simulink model "base"  (Simulink 8.7)
settings: Solver=ode1  StartTime=0.0  StopTime=inf  FixedStep=0.001  RelTol=1e-3
PostLoadFcn:
  | , if any(exist('dsrtsu_mdlpostloadfcn', 'file') == [2, 3, 6]), try dsrtsu_mdlpostloadfcn('Execute', bdroot); catch fprintf('Error in PostLoadFcn (dsrtsu_mdlpostloadfcn) for model "%s":\n %s\n', bdroot, lasterr); end, end,
libraries: rtiethernetlib x4, dsextras x1
settings Model: DSRTSU_INTERNAL_RTI_VER=480  DSRTSU_INTERNAL_RTI_TYPE=rti1007  DSRTSU_INTERNAL_RTIFPGA=70  Creator=murakami  LastModifiedBy=higo
settings DataIOCC: SignalLoggingSaveFormat=ModelDataLogs
settings OptimizationCC: BlockReduction=off  ExpressionDepthLimit=2147483647  InitFltsAndDblsToZero=on
settings DebuggingCC: AlgebraicLoopMsg=none  SaveWithParameterizedLinksMsg=none  SignalResolutionControl=TryResolveAllWithWarning  SolverPrmCheckMsg=warning  InheritedTsInSrcMsg=none  MultiTaskDSMMsg=warning  MultiTaskCondExecSysMsg=none  FcnCallInpInsideContextMsg=UseLocalSettings  UnconnectedInputMsg=none  UnconnectedOutputMsg=none  UnconnectedLineMsg=none  StateNameClashWarn=warning
settings HardwareCC: ProdLargestAtomicInteger=Integer  ProdLargestAtomicFloat=Float  ProdIntDivRoundTo=Zero  ProdEndianess=BigEndian  ProdHWDeviceType=Custom Processor->Custom  TargetIntDivRoundTo=Zero  TargetEndianess=BigEndian  TargetHWDeviceType=Custom Processor->Custom
settings RTWCC: SystemTargetFile=rti1007.tlc  MakeCommand=make_rti  TemplateMakefile=rti1007.tmf  Description=dSPACE DS1007 Hardware Platform
settings STFCustomTargetCC: ParMdlRefBuildCompliant=on  SystemTargetFile=rti1007.tlc
settings GRTTargetCC: CompOptLevelCompliant=off  ConcurrentExecutionCompliant=off  GeneratePreprocessorConditionals=Use local settings  CombineOutputUpdateFcns=off  MatFileLogging=off  CPPClassGenCompliant=off  GRTInterface=on  UseToolchainInfoCompliant=off  ExtModeMexFile=noextcomm
settings CustomProperty: DataType=RTWOptions_EnumType_C__Program Files_dSPACE RCPHIL 2016-A_MATLAB_RTI_RTI1007_TLC_rti1007_1InitialSimState  Value=RUN
settings EnumStrPairs: String=RUN

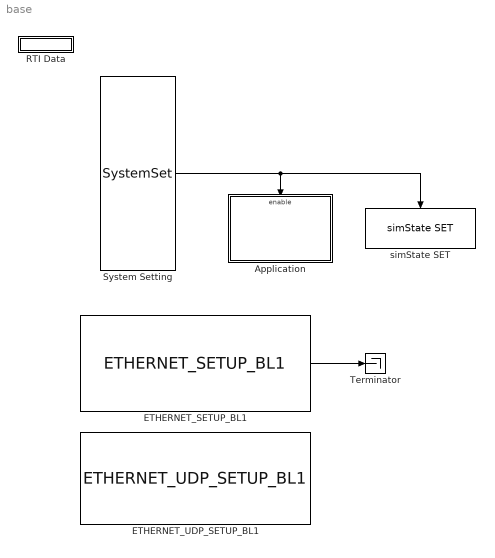
== system base ==
  Application : Subsystem  TreatAsAtomicUnit=on
  ETHERNET_SETUP_BL1 : rtiethernetlib/ETHERNET_SETUP_BL1  DSProperties=struct('RTI',struct('Version',uint32(2),'BlockType',struct('isSLSource',uint8(0),'isSLSink',uint8(0),'isHWSource',uint8(0),'isHWSink',uint8(0),'isSetup',uint8(1),'isInline',uint8(1),'isNonInline',uint8(0),'isInterrupt',uint8(0),'isChannelwise',uint8(0)),'IOBoardType','DSETHERNET','UnitType','ETHERNET','Identifier','SETUP','DialogType','ML','BlockSet','RTIETHERNET','SlaveProcessor','NONE'))  RTIBlockInterface=struct('OutputPortsWidth',int32([2 1 1 4]),'OutputPortsActive',[1 0 0 0],'OutputPortsName',{{['Link Status'],['Watchdog Status'],['DHCP Status'],['Local IP']}},'OutputPortsDataType',{{'SS_UINT32','SS_UINT32','SS_UINT32','SS_UINT8'}},'InitLevel',3,'IconTransparency','on','BlockDisplay',{{['Ethernet Setup\n\nLocal IP: 10.1.196.179'],'left'}},'DialogFcn','rtiethernetsetupgui','BlockName',struct('Token',{{'ETHERNET_SETUP_BL1'}}))  RTIBlockParameters=struct('DHCPserverMode',{{0,'OFF',[0 1]}},'LocalIpNum1',{{'10','OFF',[0 255]}},'LocalIpNum2',{{'1','OFF',[0 255]}},'LocalIpNum3',{{'196','OFF',[0 255]}},'LocalIpNum4',{{'179','OFF',[0 255]}},'SubnetMaskNum1',{{'255','OFF',[0 255]}},'SubnetMaskNum2',{{'255','OFF',[0 255]}},'SubnetMaskNum3',{{'255','OFF',[0 255]}},'SubnetMaskNum4',{{'0','OFF',[0 255]}},'GatewayNum1',{{'0','OFF',[0 255]}},'GatewayNum2',{{'0','OFF',[0 255]}},'GatewayNum3',{{'0','OFF',[0 255]}},'GatewayNum4',{{'0','OFF',[0 255]}},'LinkStatusOutPortMode',{{1,'OFF',[0 1]}},'NumOfEthConnectors',{{2,'ON',[1 16]}},'WatchdogStatusOutPortMode',{{0,'OFF',[0 1]}},'LocalIpOutPortMode',{{0,'OFF',[0 1]}},'IpAndSubmaskCheck',{{int32(1),'OFF',[0 1]}},'TLCFileName',{{'rtiethernetsetup','OFF',[]}})  RTISFcnParameters=struct('DHCPserverMode','int32','LocalIpNum1','uint8','LocalIpNum2','uint8','LocalIpNum3','uint8','LocalIpNum4','uint8','SubnetMaskNum1','uint8','SubnetMaskNum2','uint8','SubnetMaskNum3','uint8','SubnetMaskNum4','uint8','GatewayNum1','uint8','GatewayNum2','uint8','GatewayNum3','uint8','GatewayNum4','uint8','LinkStatusOutPortMode','int32','NumOfEthConnectors','int32','WatchdogStatusOutPortMode','int32','LocalIpOutPortMode','int32','TLCFileName','char')  RTIBlockParaDefault=struct('DHCPserverMode',0,'LocalIpNum1',192,'LocalIpNum2',168,'LocalIpNum3',140,'LocalIpNum4',6,'SubnetMaskNum1',255,'SubnetMaskNum2',255,'SubnetMaskNum3',255,'SubnetMaskNum4',0,'GatewayNum1',0,'GatewayNum2',0,'GatewayNum3',0,'GatewayNum4',0,'LinkStatusOutPortMode',1,'NumOfEthConnectors',3,'WatchdogStatusOutPortMode',0,'LocalIpOutPortMode',0,'IpAndSubmaskCheck',1,'TLCFileName','rtiethernetsetup')
  ETHERNET_UDP_SETUP_BL1 : rtiethernetlib/ETHERNET_UDP_SETUP_BL1  DSProperties=struct('RTI',struct('Version',uint32(2),'BlockType',struct('isSLSource',uint8(1),'isSLSink',uint8(1),'isHWSource',uint8(0),'isHWSink',uint8(0),'isSetup',uint8(0),'isInline',uint8(1),'isNonInline',uint8(0),'isInterrupt',uint8(0),'isChannelwise',uint8(0)),'IOBoardType','DSETHERNET','UnitType','UDP','Identifier','SETUPUDP','DialogType','ML','BlockSet','RTIETHERNET','SlaveProcessor','NONE'))  RTIBlockInterface=struct('OutputPortsWidth',int32(2),'OutputPortsActive',0,'OutputPortsName',{{['RX Dropped Frames']}},'OutputPortsDataType',{{'SS_DOUBLE'}},'InputPortsWidth',int32([4 1]),'InputPortsActive',int32([0 0]),'InputPortsName',{{['RX Remote IP Filter'],['RX Remote Port Filter']}},'InputPortsDataType',{{'SS_UINT8','SS_UINT16'}},'RWork',{{{'RX_DROPPED_FRAMES',uint32(2)}}},'InitLevel',3,'IconTransparency','on','BlockDisplay',{{['Ethernet UDP/IP\nSetup\n\nSocket ID: 0'],'center'}},'DialogFcn','rtiethernetsetupudpgui','BlockName',struct('Token',{{'ETHERNET_UDP_SETUP_BL1'}}))  RTIBlockParameters=struct('SocketId',{{0,'OFF',[]}},'EnableSocketBind',{{1,'OFF',[0 1]}},'AcceptAnyRxRemoteIp',{{1,'OFF',[0 1]}},'RxRemoteIpNum1',{{'10','OFF',[0 255]}},'RxRemoteIpNum2',{{'1','OFF',[0 255]}},'RxRemoteIpNum3',{{'196','OFF',[0 255]}},'RxRemoteIpNum4',{{'18','OFF',[0 255]}},'EnableDynamicRxRemoteIpFilter',{{0,'OFF',[0 1]}},'AcceptAnyRxRemotePort',{{1,'OFF',[0 1]}},'RxRemotePort',{{'49002','OFF',[1 65535]}},'EnableDynamicRxRemotePortFilter',{{0,'OFF',[0 1]}},'TxRemoteIpNum1',{{'10','OFF',[0 255]}},'TxRemoteIpNum2',{{'1','OFF',[0 255]}},'TxRemoteIpNum3',{{'196','OFF',[0 255]}},'TxRemoteIpNum4',{{'178','OFF',[0 255]}},'TxRemotePort',{{'52001','OFF',[1 65535]}},'SpecifyLocalPort',{{1,'OFF',[0 1]}},'LocalPort',{{'50006','OFF',[1 65535]}},'InterruptMode',{{0,'OFF',[0 1]}},'RxDroppedFramesOutPortMode',{{0,'OFF',[0 1]}},'RemoteIpNumCheck',{{0,'OFF',[0 1]}},'RemotePortCheck',{{0,'OFF',[0 1]}},'LocalPortCheck',{{1,'OFF',[0 1]}},'DHCPserverModeEnabled',{{0,'OFF',[0 1]}},'TLCFileName',{{'rtiethernetsetupudp','OFF',[]}})  RTISFcnParameters=struct('SocketId','double','EnableSocketBind','int32','AcceptAnyRxRemoteIp','int32','RxRemoteIpNum1','uint8','RxRemoteIpNum2','uint8','RxRemoteIpNum3','uint8','RxRemoteIpNum4','uint8','EnableDynamicRxRemoteIpFilter','int32','AcceptAnyRxRemotePort','int32','RxRemotePort','uint16','EnableDynamicRxRemotePortFilter','int32','TxRemoteIpNum1','uint8','TxRemoteIpNum2','uint8','TxRemoteIpNum3','uint8','TxRemoteIpNum4','uint8','TxRemotePort','uint16','SpecifyLocalPort','int32','LocalPort','uint16','InterruptMode','int32','RxDroppedFramesOutPortMode','int32','DHCPserverModeEnabled','int32','TLCFileName','char')  RTIBlockParaDefault=struct('SocketId',-1,'EnableSocketBind',1,'AcceptAnyRxRemoteIp',1,'RxRemoteIpNum1',0,'RxRemoteIpNum2',0,'RxRemoteIpNum3',0,'RxRemoteIpNum4',0,'EnableDynamicRxRemoteIpFilter',0,'AcceptAnyRxRemotePort',1,'RxRemotePort',49002,'EnableDynamicRxRemotePortFilter',0,'TxRemoteIpNum1',0,'TxRemoteIpNum2',0,'TxRemoteIpNum3',0,'TxRemoteIpNum4',0,'TxRemotePort',49002,'SpecifyLocalPort',0,'LocalPort',49001,'InterruptMode',0,'RxDroppedFramesOutPortMode',0,'RemoteIpNumCheck',0,'RemotePortCheck',0,'LocalPortCheck',0,'DHCPserverModeEnabled',0,'TLCFileName','rtiethernetsetupudp')
  RTI Data : Subsystem  Tag=struct('RTIDataServer',struct('RTIDataServerVs','2','RTIModelDescription','struct(''main'',''base'',''sub'','''',''isMp'',0)'))  LoadFcn="if exist('rtidc'), try,  rtidc('DataHostBlockClbLoad', gcbh); catch, disp(['Warning: ''LoadFcn'' for RTI Data block failed: ' lasterr]); end, end,"  mask(RTI_DATA_HOST){}
      mask help:
      | RTI Data Block.
      | This block is used by RTI to store internal model-dependent data.
      | Please keep this block on the root level of the model. Deleting this block will result in data loss.
      |
      | NEVER DELETE OR COPY THIS BLOCK!
      settings: CopyFcn="if exist('rtidc'), try,  rtidc('DataHostBlockClbCopy', gcbh); catch, disp(['Warning: ''CopyFcn'' for RTI Data block failed: ' lasterr]); end, end,"  DeleteFcn="if exist('rtidc'), try,  rtidc('DataHostBlockClbDelete', gcbh); catch, disp(['Warning: ''DeleteFcn'' for RTI Data block failed: ' lasterr]); end, end,"  ModelCloseFcn="if exist('rtidc'), try,  rtidc('DataHostBlockClbModelClose', gcbh); catch, disp(['Warning: ''ModelCloseFcn'' for RTI Data block failed: ' lasterr]); end, end,"  PreSaveFcn="if exist('rtidc'), try,  rtidc('DataHostBlockClbPreSave', gcbh); catch, disp(['Warning: ''PreSaveFcn'' for RTI Data block failed: ' lasterr]); end, end,"  PostSaveFcn="if exist('rtidc'), try,  rtidc('DataHostBlockClbPostSave', gcbh); catch, disp(['Warning: ''PostSaveFcn'' for RTI Data block failed: ' lasterr]); end, end,"  NameChangeFcn="if exist('rtidc'), try,  rtidc('DataHostBlockClbNameChange', gcbh); catch, disp(['Warning: ''NameChangeFcn'' for RTI Data block failed: ' lasterr]); end, end,"
      mask Help:
      | RTI Data Block.
      | This block is used by RTI to store internal model-dependent data.
      | Please keep this block on the root level of the model. Deleting this block will result in data loss.
      | 
      | NEVER DELETE OR COPY THIS BLOCK!
      mask Display:
      | text(0.5, 0.5, 'RTI Data', 'HorizontalAlignment', 'center');
      | plot([1 0]);
  System Setting : S-Function  FunctionName=SystemSet  SFunctionDeploymentMode=off  EnableBusSupport=off
  Terminator : Terminator
  simState SET : dsextras/simState SET  TriggerPort=falling  EnablePort=none  SimStateMode=STOP  TLCFileName=rti_simstate_set  Reserved1=[]  Reserved2=[]  Reserved3=[]  Reserved4=[]  DSProperties=struct('RTI',struct('Version',uint32(1),'BlockType',struct('isSLSource',uint8(1),'isSLSink',uint8(0),'isHWSource',uint8(0),'isHWSink',uint8(0),'isSetup',uint8(0),'isInline',uint8(1),'isNonInline',uint8(0),'isInterrupt',uint8(0),'isChannelwise',uint8(0)),'IOBoardType','EXTRAS','UnitType','SIMSTATESET','Identifier','SIMSTATESET','DialogType','SL','BlockSet','NONE','SlaveProcessor','NONE'))  RTIBlockInterface=struct('OutputPortsWidth',int32(0),'BlockDisplay',{{['simState STOP'],'center'}},'IconTransparency','on','InitLevel',2,'BlockName',struct('Token',{{['simState SET']}}),'TriggerPort',{{'falling'}},'EnablePort',{{'none'}},'MaskDescription',['Set simState to the specified value when the block is executed.'])  RTIBlockParameters=struct('TriggerPort',{{3,'OFF',[]}},'EnablePort',{{1,'OFF',[]}},'SimStateMode',{{3,'OFF',[]}},'TLCFileName',{{'rti_simstate_set','OFF',[]}})  RTISFcnParameters=struct('TriggerPort','double','EnablePort','double','SimStateMode','char','TLCFileName','char')  RTIBlockParaDefault=struct('TriggerPort',2,'EnablePort',1,'SimStateMode',1,'TLCFileName','rti_simstate_set')
  wires:
  ETHERNET_SETUP_BL1/1 -> Terminator/1
  System Setting/1 -> Application/Enable, simState SET/Trigger

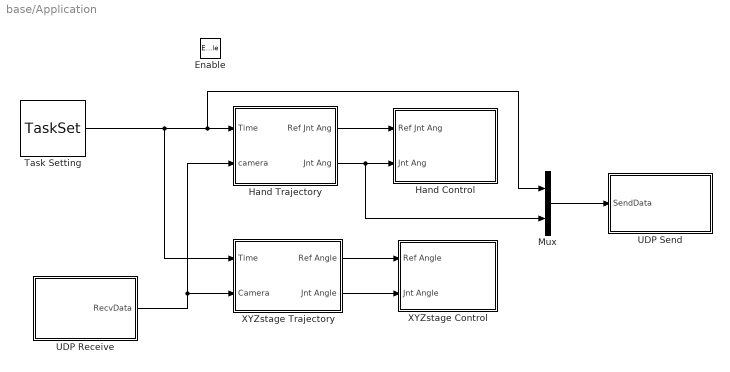
== system base/Application ==
  Enable : EnablePort  StatesWhenEnabling=reset
  Hand Control : Subsystem
  Hand Trajectory : Subsystem
  Mux : Mux  Inputs=2
  Task Setting : S-Function  FunctionName=TaskSet  SFunctionDeploymentMode=off  EnableBusSupport=off
  UDP Receive : Subsystem
  UDP Send : Subsystem
  XYZstage Control : Subsystem
  XYZstage Trajectory : Subsystem
  wires:
  Hand Trajectory/1(Ref Jnt Ang) -> Hand Control/1(Ref Jnt Ang)
  Hand Trajectory/2(Jnt Ang) -> Mux/2, Hand Control/2(Jnt Ang)
  Task Setting/1 -> XYZstage Trajectory/1(Time), Mux/1, Hand Trajectory/1(Time)
  UDP Receive/1(RecvData) -> XYZstage Trajectory/2(Camera), Hand Trajectory/2(camera)
  XYZstage Trajectory/1(Ref Angle) -> XYZstage Control/1(Ref Angle)
  XYZstage Trajectory/2(Jnt Angle) -> XYZstage Control/2(Jnt Angle)
  Mux/1 -> UDP Send/1(SendData)

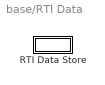
== system base/RTI Data ==
  RTI Data Store : Subsystem  Tag="struct('private',struct('version',struct('dsVer',uint32(2)),'access',struct('modified',['23-Jul-2018 20:42:30'],'type','Model','isPerm',1)),'public',struct('main',struct('data',[]),'sub',struct('name',{{'base'}},'data',{{struct('TH',struct('thTaskInfo',struct('taskType',{'TIMER','HWINT','TMRINT','SWINT','GLINT'},'tasksNumOf',{1,0,0,0,0},'srcIds',{{'TIMERA'},{},{},{},{}},'taskNames',{{['Timer Task 1']},{},{},{},{}})),'th_tc',struct('dataType','TASK','taskGroupId','','taskGroupList',{{}},'taskSchedulingPolicy','FCFS','taskType','TIMER','blkh',-1,'srcId','TIMERA','srcSgnName',['Timer A interrupt'],'srcCpuName','','taskName',['Timer Task 1  [0.001] s'],'taskNameDisplayExt','','smplTime',0.001,'smplTimeOffs',0,'hasFixedPriority',0,'priority',1,'hasFixedOvc',0,'ovcType',1,'ovcMax',1),'tc_th',struct('dataType','TASK','taskGroupId','','taskGroupList',{{}},'taskSchedulingPolicy','FCFS','taskType','TIMER','blkh',-1,'srcId','TIMERA','srcSgnName',['Timer A interrupt'],'srcCpuName','','taskName',['Timer Task 1  [0.001] s'],'taskNameDisplayExt','','smplTime',0.001,'smplTimeOffs',0,'hasFixedPriority',0,'priority',1,'hasFixedOvc',0,'ovcType',1,'ovcMax',1))}})))"  mask(RTI_DATA_STORE){}
      mask help:
      | RTI Data Store Block. This block is used by RTI to store internal model dependent data. Deleting this block will result in data loss.
      |
      | NEVER DELETE, COPY, OR MODIFY THIS BLOCK!
      mask Help:
      | RTI Data Store Block. This block is used by RTI to store internal model dependent data. Deleting this block will result in data loss.
      | 
      | NEVER DELETE, COPY, OR MODIFY THIS BLOCK!
      mask Display: text(0.5, 0.5, ' ', 'HorizontalAlignment', 'center');

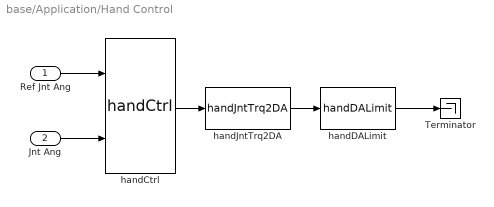
== system base/Application/Hand Control ==
  Ref Jnt Ang : Inport
  Jnt Ang : Inport  Port=2
  Terminator : Terminator
  handCtrl : S-Function  FunctionName=handCtrl  SFunctionDeploymentMode=off  EnableBusSupport=off
  handDALimit : S-Function  FunctionName=handDALimit  SFunctionDeploymentMode=off  EnableBusSupport=off
  handJntTrq2DA : S-Function  FunctionName=handJntTrq2DA  SFunctionDeploymentMode=off  EnableBusSupport=off
  wires:
  Jnt Ang/1 -> handCtrl/2
  Ref Jnt Ang/1 -> handCtrl/1
  handCtrl/1 -> handJntTrq2DA/1
  handJntTrq2DA/1 -> handDALimit/1
  handDALimit/1 -> Terminator/1

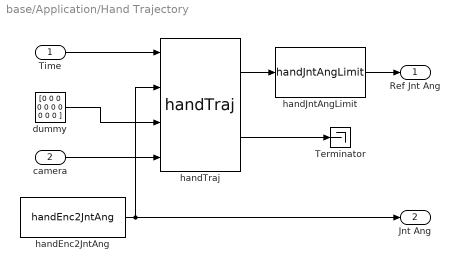
== system base/Application/Hand Trajectory ==
  Time : Inport
  camera : Inport  Port=2
  Terminator : Terminator
  dummy : Constant  Value=[0 0 0 0 0 0 0 0 0 0 ]
  handEnc2JntAng : S-Function  FunctionName=handEnc2JntAng  SFunctionDeploymentMode=off  EnableBusSupport=off
  handJntAngLimit : S-Function  FunctionName=handJntAngLimit  SFunctionDeploymentMode=off  EnableBusSupport=off
  handTraj : S-Function  FunctionName=handTraj  SFunctionDeploymentMode=off  EnableBusSupport=off
  Ref Jnt Ang : Outport
  Jnt Ang : Outport  Port=2
  wires:
  Time/1 -> handTraj/1
  handEnc2JntAng/1 -> handTraj/2, Jnt Ang/1
  handTraj/1 -> handJntAngLimit/1
  handJntAngLimit/1 -> Ref Jnt Ang/1
  handTraj/2 -> Terminator/1
  dummy/1 -> handTraj/3
  camera/1 -> handTraj/4

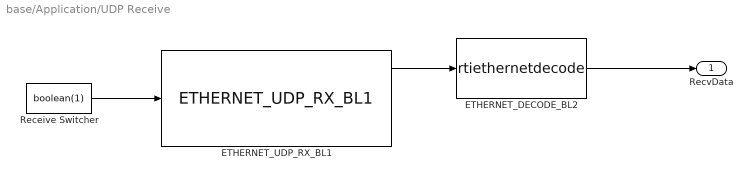
== system base/Application/UDP Receive ==
  ETHERNET_DECODE_BL2 : S-Function  FunctionName=rtiethernetdecode  Parameters=byteordering,offset,auto_offset,datatype,one_datatype,sampletime  SFunctionDeploymentMode=off  EnableBusSupport=off  mask(Ethernet Decode){byteordering=Little endian (Intel), offset=[0], auto_offset=on, datatype=9, one_datatype=on, sampletime=-1}
      mask prompts: byteordering "Byte ordering:"; offset "Offset (bytes):"; auto_offset "Auto offset"; one_datatype "One datatype only"
      mask help:
      | Converts a byte input data stream into the specified datatypes on the output port.
      |
      | Datatype codes:
      | BOOLEAN:  1   //   INT8:      2   //   UINT8:    3
      | INT16  :     4   //   UINT16:  5   //   INT32:     6
      | UINT32 :    7   //   FLOAT:    8   //   DOUBLE:  9
      mask Help: To get further information on this block, refer to the RTI Ethernet blockset documentation.
      mask TypeOptions byteordering: Big endian (Motorola) | Little endian (Intel)
      mask Callback auto_offset: rtiethernetfcnlib('EnableEnDecodeGuiControl', gcbh, 'auto_offset', 2)
      mask Display: text(0.5,0.5, 'Ethernet\nDecode', 'HorizontalAlignment', 'center')
  ETHERNET_UDP_RX_BL1 : rtiethernetlib/ETHERNET_UDP_RX_BL1  DSProperties=struct('RTI',struct('Version',uint32(1),'BlockType',struct('isSLSource',uint8(1),'isSLSink',uint8(1),'isHWSource',uint8(0),'isHWSink',uint8(1),'isSetup',uint8(0),'isInline',uint8(1),'isNonInline',uint8(0),'isInterrupt',uint8(0),'isChannelwise',uint8(0)),'IOBoardType','DSETHERNET','UnitType','UDP','Identifier','RXUDP','DialogType','ML','BlockSet','RTIETHERNET','SlaveProcessor','NONE'))  RTIBlockInterface=struct('OutputPortsWidth',int32([112 1 1 1 4 1]),'OutputPortsActive',[1 1 1 0 0 0],'OutputPortsName',{{'Data','Status',['Received Frames'],['Received Bytes'],['Remote IP'],['Remote Port']}},'OutputPortsDataType',{{'SS_UINT8','SS_UINT32','SS_DOUBLE','SS_UINT32','SS_UINT8','SS_UINT16'}},'InputPortsWidth',int32(1),'InputPortsActive',1,'InputPortsName',{{'Enable'}},'InputPortsDataType',{{'SS_BOOLEAN'}},'RWork',{{{'RECEIVED_FRAMES',uint32(1)}}},'InitLevel',3,'IconTransparency','on','BlockDisplay',{{['Ethernet UDP/IP\nRX\n\nSocket ID: 0'],'center'}},'DialogFcn','rtiethernetrxudpgui','BlockName',struct('Token',{{'ETHERNET_UDP_RX_BL1'}}))  RTIBlockParameters=struct('SocketIdIndex',{{2,'OFF',[1 2]}},'SocketId',{{0,'OFF',[-1 inf]}},'RemoteIp',{{['<NOT AVAILABLE>'],'OFF',[]}},'RemotePort',{{['<NOT AVAILABLE>'],'OFF',[]}},'LocalPort',{{50006,'OFF',[]}},'FrameSize',{{'112','OFF',[1 65507]}},'EnableVariableFrameSize',{{0,'OFF',[0 1]}},'VariableFrameSizeMode',{{1,'OFF',[1 2]}},'InterruptMode',{{0,'OFF',[0 1]}},'RemoteIpOutPortMode',{{0,'OFF',[0 1]}},'RemotePortOutPortMode',{{0,'OFF',[0 1]}},'TLCFileName',{{'rtiethernetrxudp','OFF',[]}})  RTISFcnParameters=struct('SocketIdIndex','int32','SocketId','double','FrameSize','uint16','EnableVariableFrameSize','int32','VariableFrameSizeMode','int32','InterruptMode','int32','RemoteIpOutPortMode','int32','RemotePortOutPortMode','int32','TLCFileName','char')  RTIBlockParaDefault=struct('SocketIdIndex',1,'SocketId',-1,'RemoteIp',['<NOT AVAILABLE>'],'RemotePort',['<NOT AVAILABLE>'],'LocalPort',['<NOT AVAILABLE>'],'FrameSize',1024,'EnableVariableFrameSize',0,'VariableFrameSizeMode',1,'InterruptMode',0,'RemoteIpOutPortMode',0,'RemotePortOutPortMode',0,'TLCFileName','rtiethernetrxudp')
  Receive Switcher : Constant  Value=boolean(1)
  RecvData : Outport
  wires:
  ETHERNET_DECODE_BL2/1 -> RecvData/1
  ETHERNET_UDP_RX_BL1/1 -> ETHERNET_DECODE_BL2/1
  Receive Switcher/1 -> ETHERNET_UDP_RX_BL1/1

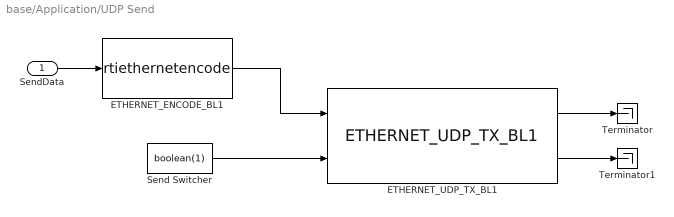
== system base/Application/UDP Send ==
  SendData : Inport
  ETHERNET_ENCODE_BL1 : S-Function  FunctionName=rtiethernetencode  Parameters=byteordering,offset,auto_offset,datatype,one_datatype,sampletime  SFunctionDeploymentMode=off  EnableBusSupport=off  mask(Ethernet Encode){byteordering=Little endian (Intel), offset=[0], auto_offset=on, datatype=9, one_datatype=on, sampletime=-1}
      mask prompts: byteordering "Byte ordering:"; offset "Offset (bytes):"; auto_offset "Auto offset"; one_datatype "One datatype only"
      mask help:
      | Converts an input signal consisting of datatypes into a byte data stream on the output port.
      |
      | Datatype codes:
      | BOOLEAN:  1   //   INT8:      2   //   UINT8:    3
      | INT16  :     4   //   UINT16:  5   //   INT32:     6
      | UINT32 :    7   //   FLOAT:    8   //   DOUBLE:  9
      mask Help: To get further information on this block, refer to the RTI Ethernet blockset documentation.
      mask TypeOptions byteordering: Big endian (Motorola) | Little endian (Intel)
      mask Callback auto_offset: rtiethernetfcnlib('EnableEnDecodeGuiControl', gcbh, 'auto_offset', 2)
      mask Display: text(0.5,0.5, 'Ethernet\nEncode', 'HorizontalAlignment', 'center')
  ETHERNET_UDP_TX_BL1 : rtiethernetlib/ETHERNET_UDP_TX_BL1  DSProperties=struct('RTI',struct('Version',uint32(1),'BlockType',struct('isSLSource',uint8(1),'isSLSink',uint8(1),'isHWSource',uint8(0),'isHWSink',uint8(1),'isSetup',uint8(0),'isInline',uint8(1),'isNonInline',uint8(0),'isInterrupt',uint8(0),'isChannelwise',uint8(0)),'IOBoardType','DSETHERNET','UnitType','UDP','Identifier','TXUDP','DialogType','ML','BlockSet','RTIETHERNET','SlaveProcessor','NONE'))  RTIBlockInterface=struct('OutputPortsWidth',int32([1 1]),'OutputPortsActive',[1 1],'OutputPortsName',{{'Status',['Sent Frames']}},'OutputPortsDataType',{{'SS_UINT32','SS_DOUBLE'}},'InputPortsWidth',int32([96 1 1 4 1]),'InputPortsActive',[1 1 0 0 0],'InputPortsName',{{'Data','Enable',['Bytes to Send'],['Remote IP'],['Remote Port']}},'InputPortsDataType',{{'SS_UINT8','SS_BOOLEAN','SS_UINT32','SS_UINT8','SS_UINT16'}},'RWork',{{{'SENT_FRAMES',uint32(1)}}},'InitLevel',3,'IconTransparency','on','BlockDisplay',{{['Ethernet UDP/IP\nTX\n\nSocket ID: 0'],'center'}},'DialogFcn','rtiethernettxudpgui','BlockName',struct('Token',{{'ETHERNET_UDP_TX_BL1'}}))  RTIBlockParameters=struct('SocketIdIndex',{{2,'OFF',[1 2]}},'SocketId',{{0,'OFF',[-1 inf]}},'RemoteIp',{{'10.1.196.178','OFF',[]}},'RemotePort',{{52001,'OFF',[]}},'LocalPort',{{50006,'OFF',[]}},'EnableDynamicRemoteIp',{{0,'OFF',[0 1]}},'EnableDynamicRemotePort',{{0,'OFF',[0 1]}},'FrameSize',{{'96','OFF',[1 65507]}},'EnableVariableFrameSize',{{0,'OFF',[0 1]}},'SentFramesOutPortMode',{{1,'OFF',[0 1]}},'RemoteIpNum',{{[10 1 196 178],'OFF',[0 255]}},'RemotePortNum',{{52001,'OFF',[0 65535]}},'TLCFileName',{{'rtiethernettxudp','OFF',[]}})  RTISFcnParameters=struct('SocketIdIndex','int32','SocketId','double','EnableDynamicRemoteIp','int32','EnableDynamicRemotePort','int32','FrameSize','uint16','EnableVariableFrameSize','int32','SentFramesOutPortMode','int32','RemoteIpNum','uint8','RemotePortNum','uint16','TLCFileName','char')  RTIBlockParaDefault=struct('SocketIdIndex',1,'SocketId',-1,'RemoteIp',['<NOT AVAILABLE>'],'RemotePort',['<NOT AVAILABLE>'],'LocalPort',['<NOT AVAILABLE>'],'EnableDynamicRemoteIp',0,'EnableDynamicRemotePort',0,'FrameSize',1024,'EnableVariableFrameSize',0,'SentFramesOutPortMode',1,'RemoteIpNum',[0 0 0 0],'RemotePortNum',0,'TLCFileName','rtiethernettxudp')
  Send Switcher : Constant  Value=boolean(1)
  Terminator : Terminator
  Terminator1 : Terminator
  wires:
  Send Switcher/1 -> ETHERNET_UDP_TX_BL1/2
  ETHERNET_UDP_TX_BL1/1 -> Terminator/1
  ETHERNET_UDP_TX_BL1/2 -> Terminator1/1
  ETHERNET_ENCODE_BL1/1 -> ETHERNET_UDP_TX_BL1/1
  SendData/1 -> ETHERNET_ENCODE_BL1/1

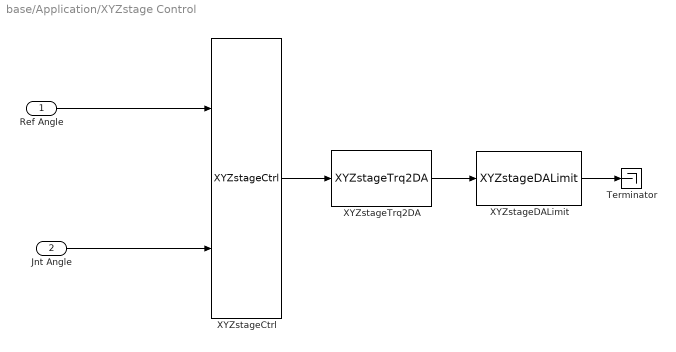
== system base/Application/XYZstage Control ==
  Ref Angle : Inport
  Jnt Angle : Inport  Port=2
  Terminator : Terminator
  XYZstageCtrl : S-Function  FunctionName=XYZstageCtrl  SFunctionDeploymentMode=off  EnableBusSupport=off
  XYZstageDALimit : S-Function  FunctionName=XYZstageDALimit  SFunctionDeploymentMode=off  EnableBusSupport=off
  XYZstageTrq2DA : S-Function  FunctionName=XYZstageTrq2DA  SFunctionDeploymentMode=off  EnableBusSupport=off
  wires:
  Jnt Angle/1 -> XYZstageCtrl/2
  Ref Angle/1 -> XYZstageCtrl/1
  XYZstageCtrl/1 -> XYZstageTrq2DA/1
  XYZstageDALimit/1 -> Terminator/1
  XYZstageTrq2DA/1 -> XYZstageDALimit/1

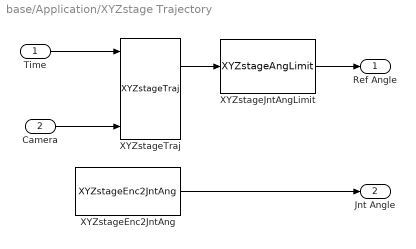
== system base/Application/XYZstage Trajectory ==
  Time : Inport
  Camera : Inport  Port=2
  XYZstageEnc2JntAng : S-Function  FunctionName=XYZstageEnc2JntAng  SFunctionDeploymentMode=off  EnableBusSupport=off
  XYZstageJntAngLimit : S-Function  FunctionName=XYZstageAngLimit  SFunctionDeploymentMode=off  EnableBusSupport=off
  XYZstageTraj : S-Function  FunctionName=XYZstageTraj  SFunctionDeploymentMode=off  EnableBusSupport=off
  Ref Angle : Outport
  Jnt Angle : Outport  Port=2
  wires:
  XYZstageJntAngLimit/1 -> Ref Angle/1
  Time/1 -> XYZstageTraj/1
  XYZstageTraj/1 -> XYZstageJntAngLimit/1
  Camera/1 -> XYZstageTraj/4
  XYZstageEnc2JntAng/1 -> Jnt Angle/1

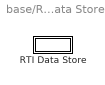
== system base/RTI Data/RTI Data Store ==
  RTI Data Store : Subsystem  mask(RTI_DATA_STORE){}
      mask help:
      | RTI Data Store Block. This block is used by RTI to store internal model dependent data. Deleting this block will result in data loss.
      |
      | NEVER DELETE, COPY, OR MODIFY THIS BLOCK!
      mask Help:
      | RTI Data Store Block. This block is used by RTI to store internal model dependent data. Deleting this block will result in data loss.
      | 
      | NEVER DELETE, COPY, OR MODIFY THIS BLOCK!
      mask Display: text(0.5, 0.5, ' ', 'HorizontalAlignment', 'center');

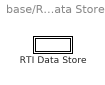
== system base/RTI Data/RTI Data Store/RTI Data Store ==
  RTI Data Store : Subsystem  mask(RTI_DATA_STORE){}
      mask help:
      | RTI Data Store Block. This block is used by RTI to store internal model dependent data. Deleting this block will result in data loss.
      |
      | NEVER DELETE, COPY, OR MODIFY THIS BLOCK!
      mask Help:
      | RTI Data Store Block. This block is used by RTI to store internal model dependent data. Deleting this block will result in data loss.
      | 
      | NEVER DELETE, COPY, OR MODIFY THIS BLOCK!
      mask Display: text(0.5, 0.5, ' ', 'HorizontalAlignment', 'center');

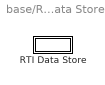
== system base/RTI Data/RTI Data Store/RTI Data Store/RTI Data Store ==
  RTI Data Store : Subsystem  mask(RTI_DATA_STORE){}
      mask help:
      | RTI Data Store Block. This block is used by RTI to store internal model dependent data. Deleting this block will result in data loss.
      |
      | NEVER DELETE, COPY, OR MODIFY THIS BLOCK!
      mask Help:
      | RTI Data Store Block. This block is used by RTI to store internal model dependent data. Deleting this block will result in data loss.
      | 
      | NEVER DELETE, COPY, OR MODIFY THIS BLOCK!
      mask Display: text(0.5, 0.5, ' ', 'HorizontalAlignment', 'center');

== system base/RTI Data/RTI Data Store/RTI Data Store/RTI Data Store/RTI Data Store ==
